simulink model "Matlab_Mission_Manager_SIM"  (R2025b)
settings: Solver=FixedStepDiscrete  StartTime=0.0  StopTime=tspan  FixedStep=dt_sim  RelTol=rel_tol  AbsTol=abs_tol
undefined symbols (not defined in the file): Cimub, const_voltage, dt_control, dt_data, dt_dvl_drr, dt_dvl_vr, dvl, initial_joystick_mode_enabled_flag, use_true_state_flag
libraries: mspsensorlib x1
settings Model: Creator=koryh  LastModifiedBy=kjhaydon

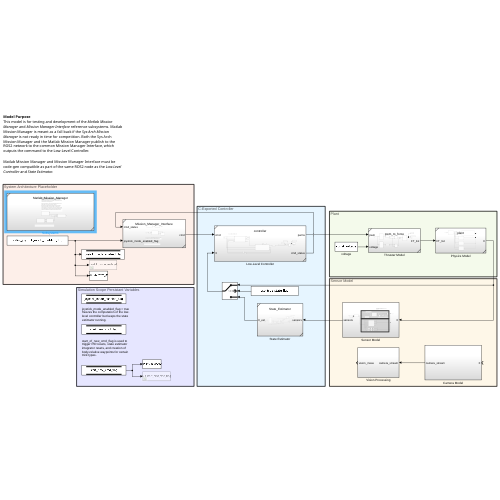
[thumbnail: Simulink's stored preview of the top-level diagram]
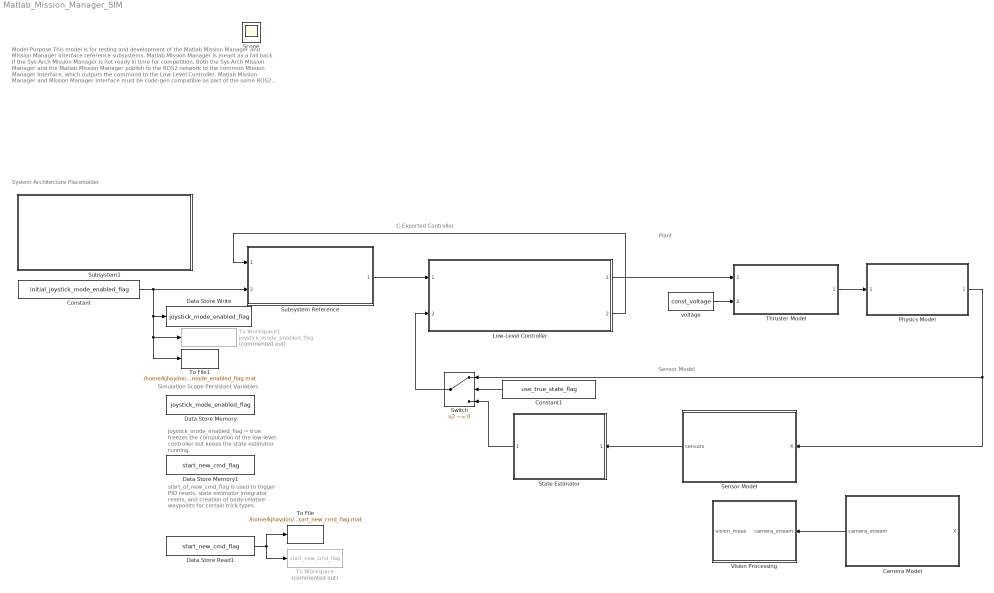
== system Matlab_Mission_Manager_SIM ==
  note: Model Purpose
      | This model is for testing and development of the Matlab Mission Manager and Mission Manager Interface reference subsystems. Matlab Mission Manager is meant as a fall back if the Sys-Arch Mission Manager is not ready in time for competition. Both the Sys Arch Mission Manager and the Matlab Mission Manager publish to the ROS2 network to the common Mission Manager Interface, which outputs the command to the Low-Level Controller.
      |
      | Matlab Mission Manager and Mission Manager Interface must be code-gen compatible as part of the same ROS2 node as the Low-Level Controller and State Estimator.
  note: joystick_mode_enabled_flag = true freezes the computation of the low-level controller but keeps the state estimator running.
  note: Simulation Scope Persistant Variables
  note: System Architecture Placeholder
  note: Sensor Model
  note: Plant
  note: C-Exported Controller
  note: start_of_new_cmd_flag is used to trigger PID resets, state estimator integrator resets, and creation of body-relative waypoints for certain trick types.
  Camera Model : Subsystem
  Constant : Constant  Value=initial_joystick_mode_enabled_flag
  Constant1 : Constant  Value=use_true_state_flag
  Data Store Memory : DataStoreMemory  DataStoreName=joystick_mode_enabled_flag  WriteAfterWriteMsg=warning  InitialValue=initial_joystick_mode_enabled_flag  ShowAdditionalParam=off  OutDataTypeStr=boolean
  Data Store Memory1 : DataStoreMemory  DataStoreName=start_new_cmd_flag  WriteAfterWriteMsg=warning  InitialValue=true  ShowAdditionalParam=off  OutDataTypeStr=boolean
  Data Store Read1 : DataStoreRead  DataStoreName=start_new_cmd_flag  IndexOptions=Index vector (dialog)  Indices=1  OutputSizes=1
  Data Store Write : DataStoreWrite  DataStoreName=joystick_mode_enabled_flag  IndexOptions=Index vector (dialog)  Indices=1  OutputSizes=1
  Low-Level Controller : Subsystem  ReferencedSubsystem=controller
  Physics Model : Subsystem  ReferencedSubsystem=plant
  Sensor Model : Subsystem
  State Estimator : Subsystem  ReferencedSubsystem=State_Estimator
  Subsystem Reference : Subsystem  ReferencedSubsystem=Mission_Manager_Interface
  Subsystem1 : Subsystem  ReferencedSubsystem=Matlab_Mission_Manager
  Switch : Switch  Criteria=u2 ~= 0  SaturateOnIntegerOverflow=off  InputSameDT=off
  Thruster Model : Subsystem  ReferencedSubsystem=pwm_to_force
  To File : ToFile  Filename=/home/kjhaydon/Github/Robosub/SimulinkPlant/data/2026_05_30_16_31_18/start_new_cmd_flag.mat  MatrixName=start_new_cmd_flag  SaveFormat=Timeseries
  To File1 : ToFile  Filename=/home/kjhaydon/Github/Robosub/SimulinkPlant/data/2026_05_30_16_31_18/joystick_mode_enabled_flag.mat  MatrixName=joystick_mode_enabled_flag  SaveFormat=Timeseries  SampleTime=dt_data
  To Workspace : ToWorkspace  Commented=on  VariableName=start_new_cmd_flag  SaveFormat=Timeseries  SampleTime=dt_data
  To Workspace1 : ToWorkspace  Commented=on  VariableName=joystick_mode_enabled_flag  SaveFormat=Timeseries  SampleTime=dt_data
  Vision Processing : Subsystem
  voltage : Constant  Value=const_voltage
  Scope : Scope
      settings: ActiveDisplayYMinimum=-0.048832566475369238  ActiveDisplayYMaximum=0.79721663606048965
  wires:
  voltage/1 -> Thruster Model/2
  Low-Level Controller/1 -> Thruster Model/1
  Thruster Model/1 -> Physics Model/1
  Subsystem Reference/1 -> Low-Level Controller/1
  Low-Level Controller/2 -> Subsystem Reference/1
  Physics Model/1 -> Sensor Model/1(X), Switch/1
  Camera Model/1(camera_stream) -> Vision Processing/1(camera_stream)
  Sensor Model/1(sensors) -> State Estimator/1
  Switch/1 -> Low-Level Controller/2
  Constant1/1 -> Switch/2
  State Estimator/1 -> Switch/3
  Data Store Read1/1 -> To File/1, To Workspace/1
  Constant/1 -> Subsystem Reference/2, To File1/1, To Workspace1/1, Data Store Write/1

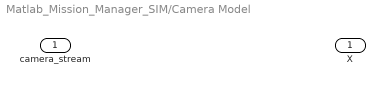
== system Matlab_Mission_Manager_SIM/Camera Model ==
  X : Inport
  camera_stream : Outport

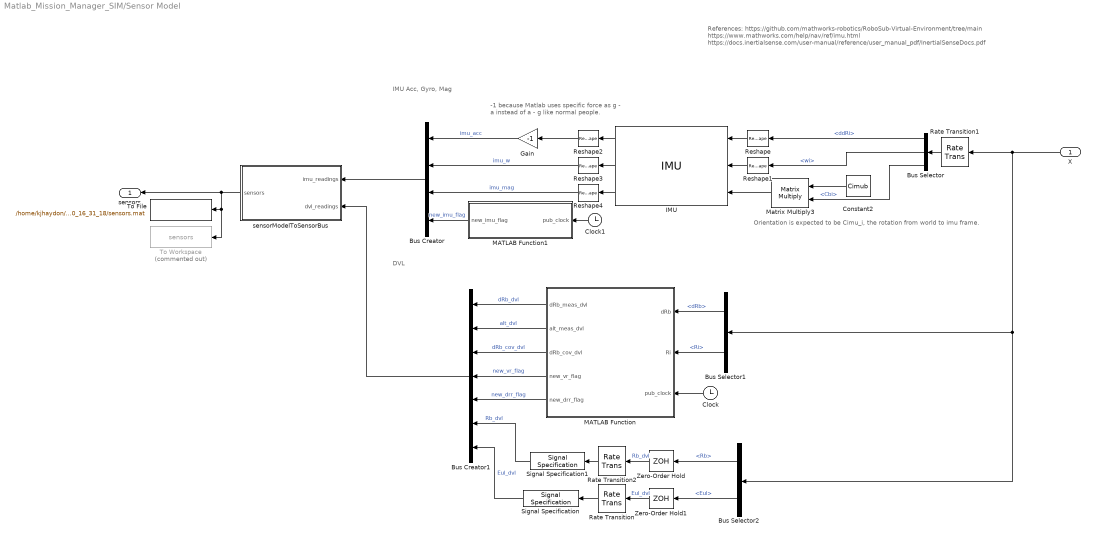
== system Matlab_Mission_Manager_SIM/Sensor Model ==
  note: IMU Acc, Gyro, Mag
  note: -1 because Matlab uses specific force as
      |  g - a instead of a - g like normal people.
  note: Orientation is expected to be Cimu_i, the rotation from world to imu frame.
  note: References:
      | https://github.com/mathworks-robotics/RoboSub-Virtual-Environment/tree/main
      | https://www.mathworks.com/help/nav/ref/imu.html
      | https://docs.inertialsense.com/user-manual/reference/user_manual_pdf/InertialSenseDocs.pdf
  note: DVL
  X : Inport  OutDataTypeStr=Bus: X_bus  SampleTime=dt_control
  Bus Creator : BusCreator  Inputs=4  OutDataTypeStr=Bus: imu_bus
  Bus Creator1 : BusCreator  Inputs=7  OutDataTypeStr=Bus: dvl_bus
  Bus Selector : BusSelector  OutputSignals=ddRi,wi,Cbi
  Bus Selector1 : BusSelector  OutputSignals=dRb,Ri
  Bus Selector2 : BusSelector  OutputSignals=Rb,Eul
  Clock : Clock
  Clock1 : Clock
  Constant2 : Constant  Value=Cimub
  Gain : Gain  Gain=-1
  IMU : mspsensorlib/IMU  DispRefFrame=NED  TemperaturePort=off  Temperature=imu.T  MagneticFieldPort=off  MagneticFieldNED=imu.Bi  MagneticFieldENU=[ -2.4169, 27.5550, 16.0849 ]  SeedDouble=67  SimulateUsing=Interpreted execution  AccelParamsMeasurementRange=imu.acc.meas_range  AccelParamsResolution=imu.acc.res  AccelParamsConstantBias=imu.acc.const_bias  AccelParamsAxesMisalignment=imu.acc.axes_skew  AccelParamsNoiseDensity=imu.acc.vel_rand_walk  AccelParamsBiasInstability=imu.acc.bias_inst  AccelParamsBiasInstabilityNumerator=imu.acc.bias_inst_num_coeffs  AccelParamsBiasInstabilityDenominator=imu.acc.bias_inst_den_coeffs  AccelParamsRandomWalk=imu.acc.acc_rand_walk  AccelParamsNoiseType=double-sided  AccelParamsTemperatureBias=imu.acc.temp_bias  AccelParamsTemperatureScaleFactor=imu.acc.temp_scale_factor  GyroParamsMeasurementRange=imu.gyro.max_read  GyroParamsResolution=imu.gyro.res  GyroParamsConstantBias=imu.gyro.const_bias  GyroParamsAxesMisalignment=imu.gyro.axes_skew  GyroParamsAccelerationBias=imu.gyro.bias_from_acc  GyroParamsNoiseDensity=imu.gyro.angle_rand_walk  GyroParamsBiasInstability=imu.gyro.bias_inst  GyroParamsBiasInstabilityNumerator=imu.gyro.bias_inst_filter_num_coeffs  GyroParamsBiasInstabilityDenominator=imu.gyro.bias_inst_filter_den_coeffs  GyroParamsRandomWalk=imu.gyro.rate_rand_walk  GyroParamsNoiseType=double-sided  GyroParamsTemperatureBias=imu.gyro.temp_bias  GyroParamsTemperatureScaleFactor=imu.gyro.temp_scale_factor  MagParamsMeasurementRange=imu.mag.max_read  MagParamsResolution=imu.mag.res  MagParamsConstantBias=imu.mag.const_bias  MagParamsAxesMisalignment=imu.mag.axes_skew  MagParamsNoiseDensity=imu.mag.white_noise_psd  MagParamsBiasInstability=imu.mag.bias_inst  MagParamsBiasInstabilityNumerator=imu.mag.bias_inst_filter_num_coeffs  MagParamsBiasInstabilityDenominator=imu.mag.bias_isnt_filter_den_coeffs  MagParamsRandomWalk=imu.mag.rand_walk  MagParamsNoiseType=double-sided  MagParamsTemperatureBias=imu.mag.temp_bias  MagParamsTemperatureScaleFactor=imu.mag.temp_scale_factor
  MATLAB Function : MATLAB Function  TreatAsAtomicUnit=on
  MATLAB Function1 : MATLAB Function  TreatAsAtomicUnit=on
  Matrix Multiply3 : Product  Multiplication=Matrix(*)
  Rate Transition : RateTransition  Deterministic=off  OutPortSampleTime=dt_control
  Rate Transition1 : RateTransition  OutPortSampleTime=dt_imu
  Rate Transition2 : RateTransition  Deterministic=off  OutPortSampleTime=dt_control
  Reshape : Reshape  OutputDimensionality=Row vector (2-D)
  Reshape1 : Reshape  OutputDimensionality=Row vector (2-D)
  Reshape2 : Reshape  OutputDimensionality=Column vector (2-D)
  Reshape3 : Reshape  OutputDimensionality=Column vector (2-D)
  Reshape4 : Reshape  OutputDimensionality=Column vector (2-D)
  Signal Specification : SignalSpecification  SampleTime=dt_control
  Signal Specification1 : SignalSpecification  SampleTime=dt_control
  To File : ToFile  Filename=/home/kjhaydon/Github/Robosub/SimulinkPlant/data/2026_05_30_16_31_18/sensors.mat  MatrixName=sensors  SaveFormat=Timeseries  SampleTime=dt_data
  To Workspace : ToWorkspace  Commented=on  VariableName=sensors  SaveFormat=Timeseries  SampleTime=dt_data
  Zero-Order Hold : ZeroOrderHold  SampleTime=dt_dvl_drr
  Zero-Order Hold1 : ZeroOrderHold  SampleTime=dt_dvl_drr
  sensorModelToSensorBus : MATLAB Function  TreatAsAtomicUnit=on
  sensors : Outport  OutDataTypeStr=Bus: sensor_bus  SampleTime=dt_control
  wires:
  X/1 -> Rate Transition1/1, Bus Selector2/1, Bus Selector1/1
  Reshape/1 -> IMU/1
  Bus Selector/2 -> Reshape1/1  "<wi>"
  IMU/1 -> Reshape2/1
  IMU/2 -> Reshape3/1
  IMU/3 -> Reshape4/1
  Reshape1/1 -> IMU/2
  Bus Selector/1 -> Reshape/1  "<ddRi>"
  Matrix Multiply3/1 -> IMU/3
  Constant2/1 -> Matrix Multiply3/1
  Bus Selector/3 -> Matrix Multiply3/2  "<Cbi>"
  Reshape2/1 -> Gain/1
  Bus Selector1/1 -> MATLAB Function/1(dRb)  "<dRb>"
  Bus Selector1/2 -> MATLAB Function/2(Ri)  "<Ri>"
  Bus Selector2/1 -> Zero-Order Hold/1  "<Rb>"
  sensorModelToSensorBus/1(sensors) -> sensors/1, To Workspace/1, To File/1
  Bus Selector2/2 -> Zero-Order Hold1/1  "<Eul>"
  Rate Transition1/1 -> Bus Selector/1
  Clock/1 -> MATLAB Function/3(pub_clock)
  Clock1/1 -> MATLAB Function1/1(pub_clock)
  Gain/1 -> Bus Creator/1  "imu_acc"
  Reshape3/1 -> Bus Creator/2  "imu_w"
  Reshape4/1 -> Bus Creator/3  "imu_mag"
  MATLAB Function1/1(new_imu_flag) -> Bus Creator/4  "new_imu_flag"
  MATLAB Function/1(dRb_meas_dvl) -> Bus Creator1/1  "dRb_dvl"
  MATLAB Function/2(alt_meas_dvl) -> Bus Creator1/2  "alt_dvl"
  MATLAB Function/3(dRb_cov_dvl) -> Bus Creator1/3  "dRb_cov_dvl"
  MATLAB Function/4(new_vr_flag) -> Bus Creator1/4  "new_vr_flag"
  MATLAB Function/5(new_drr_flag) -> Bus Creator1/5  "new_drr_flag"
  Bus Creator/1 -> sensorModelToSensorBus/1(imu_readings)
  Bus Creator1/1 -> sensorModelToSensorBus/2(dvl_readings)
  Zero-Order Hold/1 -> Rate Transition2/1  "Rb_dvl"
  Signal Specification1/1 -> Bus Creator1/6  "Rb_dvl"
  Signal Specification/1 -> Bus Creator1/7  "Eul_dvl"
  Rate Transition/1 -> Signal Specification/1
  Rate Transition2/1 -> Signal Specification1/1
  Zero-Order Hold1/1 -> Rate Transition/1  "Eul_dvl"

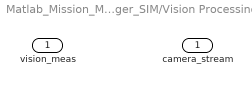
== system Matlab_Mission_Manager_SIM/Vision Processing ==
  camera_stream : Inport
  vision_meas : Outport

== matlab function Matlab_Mission_Manager_SIM/Sensor Model/MATLAB Function1 ==
  settings: updateMethod=DISCRETE  sampleTime=dt_control
  data: pub_clock input; new_imu_flag output; dt_imu parameter
function new_imu_flag = fcn(pub_clock, dt_imu)

persistent last_imu_time

if(isempty(last_imu_time))
    last_imu_time = pub_clock;
end


time_since_last_imu = pub_clock - last_imu_time;

if(time_since_last_imu < dt_imu)
    new_imu_flag = 0;
else
    new_imu_flag = 1;
    last_imu_time = pub_clock;
end

== matlab function Matlab_Mission_Manager_SIM/Sensor Model/MATLAB Function ==
  settings: updateMethod=DISCRETE  sampleTime=dt_control
  data: dRb input; dRb_meas_dvl output; Ri input; alt_meas_dvl output; dRb_cov_dvl output; dvl parameter; pub_clock input; new_vr_flag output; new_drr_flag output; dt_dvl_vr parameter; dt_dvl_drr parameter
function [dRb_meas_dvl, alt_meas_dvl, dRb_cov_dvl, new_vr_flag, new_drr_flag] = dvl_sim(dRb, Ri,dvl, pub_clock, dt_dvl_vr, dt_dvl_drr)
%{
Model from this repository:
https://github.com/mathworks-robotics/RoboSub-Virtual-Environment/
Need to modify this to give erroneous or no reading when ground lock is
available.

Also need to add noise to the altitude measurement and determine if it
needs modification based on attitude.
%}

persistent last_drr_time
persistent last_vr_time

if(isempty(last_drr_time))
    last_drr_time = pub_clock;
end
if(isempty(last_vr_time))
    last_vr_time = pub_clock;
end

time_since_last_drr = pub_clock - last_drr_time;
time_since_last_vr = pub_clock - last_vr_time;
if(time_since_last_drr < dt_dvl_drr)
    new_drr_flag = 0;
else
    new_drr_flag = 1;
    last_drr_time = pub_clock;
end
if(time_since_last_vr < dt_dvl_vr)
    new_vr_flag = 0;
else
    new_vr_flag = 1;
    last_vr_time = pub_clock;
end



%get altitude (assumes Ri is measured from the robot's starting depth
true_depth = dvl.start_depth + Ri(3); 
true_alt = dvl.pool_depth - true_depth;
alt_meas_dvl = true_alt;

%bias for velocity measurements
persistent bias
if isempty(bias)
    bias = zeros(3,1);
end


% ---------------- Update bias (Gauss-Markov) ----------------
if dvl.bias_tau > 0 && dvl.bias_sigma_ss > 0
    % Discrete-time OU: b_{k+1} = (1 - dt/tau) b_k + sqrt(2*sigma^2*dt/tau) * w
    a = max(0.0, 1.0 - dvl.bias_dt/dvl.bias_tau);
    q = sqrt(max(0.0, 2.0*dvl.bias_sigma_ss^2*dvl.bias_dt/dvl.bias_tau));
    bias = a*bias + q * randn(3,1);
else
    bias = zeros(3,1);
end

% ---------------- Add noise & bias ----------------
noise = dvl.noise_sigma .* randn(3,1);    % white noise
dRb_meas_dvl = dRb + bias + noise;

dRb_cov_dvl = diag([dvl.noise_sigma].^2);

== matlab function Matlab_Mission_Manager_SIM/Sensor Model/sensorModelToSensorBus ==
  settings: updateMethod=DISCRETE  sampleTime=dt_control
  data: imu_readings input; sensors output Bus: sensor_bus; dvl_readings input
function sensors = fcn(imu_readings, dvl_readings)

sensors = sensorModelToSensorBus(imu_readings, dvl_readings);
